simulink model "OpenFAST_ROSCO_LDP_FFP_with_FFIPC"  (R2024b)
settings: Solver=ode4  StartTime=0.0  StopTime=TMax  FixedStep=DT  RelTol=1e-3
values from neighbouring files (symbols this model uses):
  IPC = []    [HVFF_SimulinkFFIPC.m]    (also in RunExample_Simulink.m; VerticalGain_BruteForce.m)
  P = ReadWrite_FAST(fast)    [HVFF_SimulinkFFIPC.m]    (also in RunExample_Simulink.m; VerticalGain_BruteForce.m)
  verticalShear = 0.02    [HVFF_SimulinkFFIPC.m]    (also in RunExample_Simulink.m = 0.0167; VerticalGain_BruteForce.m = 0.0167)
undefined symbols (not defined in the file or in its folder): dspblkCoreblockFVToolHelper, F, gcbh, GetFASTPar, LDP, OutList, R, simu, strmatch
libraries: simulink_extras x4, simulink x3
settings Model: LastModifiedBy=demit
settings OptimizationCC: BlockReduction=off  BooleanDataType=off
settings DebuggingCC: SaveWithParameterizedLinksMsg=none  UnderspecifiedInitializationDetection=Classic  MergeDetectMultiDrivingBlocksExec=none  SignalResolutionControl=TryResolveAllWithWarning  UnconnectedInputMsg=warning  UnconnectedOutputMsg=warning  UnconnectedLineMsg=warning
settings HardwareCC: TargetUnknown=on
settings ModelReferenceCC: EnableRefExpFcnMdlSchedulingChecks=on  PropagateSignalLabelsOutOfModel=off
settings RTWCC: GPUComputeCapability=3.5  DLArmComputeVersion=19.05

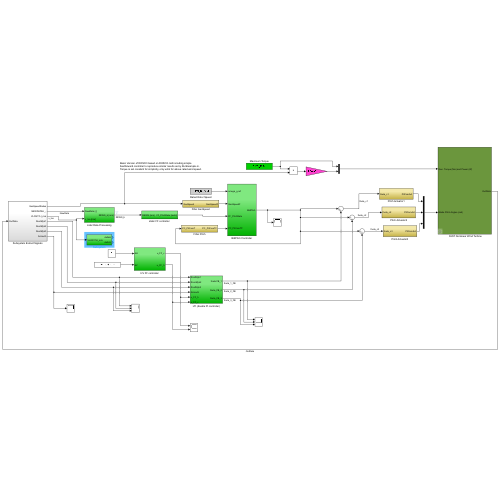
[thumbnail: Simulink's stored preview of the top-level diagram]
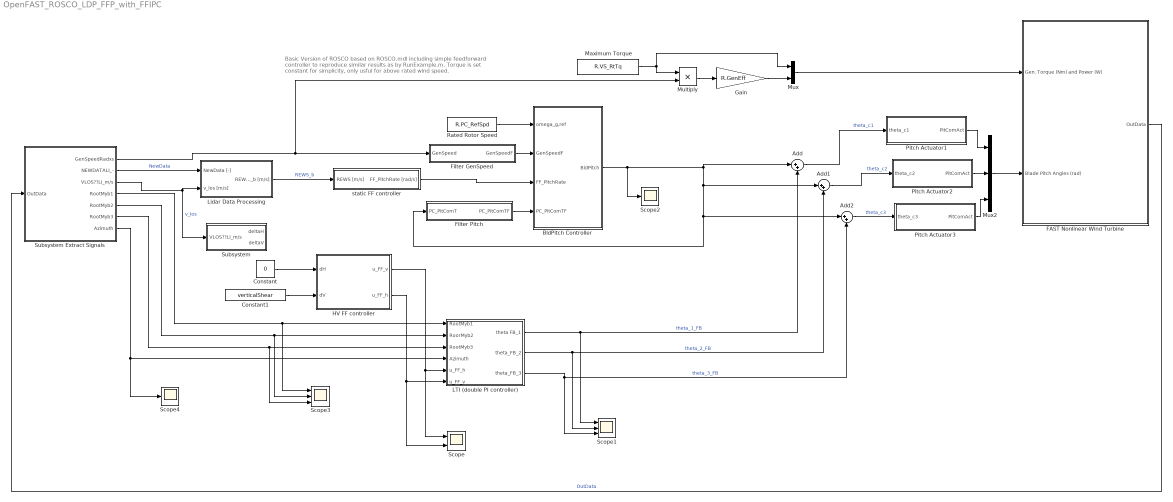
== system OpenFAST_ROSCO_LDP_FFP_with_FFIPC ==
  note: Basic Version of ROSCO based on ROSCO.mdl including simple feedforward controller to reproduce similar results as by RunExample.m.
      | Torque is set constant for simplicity, only usful for above rated wind speed.
  "  FAST Nonlinear Wind Turbine" : Subsystem  mask(FAST Nonlinear Wind Turbine){}
      mask help: This block contains the FAST S-Function.
      mask init:
      | clear FAST_SFunc
  Add : Sum  Inputs=|++
  Add1 : Sum  Inputs=|++
  Add2 : Sum  Inputs=|++
  BldPitch Controller : Subsystem
  Constant : Constant  Value=0
  Constant1 : Constant  Value=verticalShear
  Filter GenSpeed : Subsystem
  Filter Pitch : Subsystem
  Gain : Gain  Gain=R.GenEff
  HV FF controller : Subsystem
  LTI (double PI controller) : Subsystem
  Lidar Data Processing : Subsystem
  Maximum Torque : Constant  Value=R.VS_RtTq
  Multiply : Product
  Mux : Mux  Inputs=2
  Mux2 : Mux  Inputs=3
  Pitch Actuator1 : Subsystem
  Pitch Actuator2 : Subsystem
  Pitch Actuator3 : Subsystem
  Rated Rotor Speed : Constant  Value=R.PC_RefSpd
  Scope : Scope  NumInputPorts=2
  Scope1 : Scope  NumInputPorts=3
  Scope2 : Scope
  Scope3 : Scope  NumInputPorts=3
  Scope4 : Scope
  Subsystem : Subsystem
  Subsystem Extract Signals : Subsystem
  "static FF controller " : Subsystem
  wires:
  Mux2/1 -> "  FAST Nonlinear Wind Turbine"/2(Blade Pitch Angles (rad))
  BldPitch Controller/1(BldPitch) -> Scope2/1, Add/1, Add1/1, Add2/1, Filter Pitch/1(PC_PitComT)
  Rated Rotor Speed/1 -> BldPitch Controller/1(omega_g,ref)
  Subsystem Extract Signals/1(GenSpeedRadxs) -> Filter GenSpeed/1(GenSpeed), Multiply/2
  Maximum Torque/1 -> Mux/1, Multiply/1
  Filter GenSpeed/1(GenSpeedF) -> BldPitch Controller/2(GenSpeedF)
  Gain/1 -> Mux/2
  Mux/1 -> "  FAST Nonlinear Wind Turbine"/1(Gen. Torque (Nm) and Power (W))
  Multiply/1 -> Gain/1
  "  FAST Nonlinear Wind Turbine"/1(OutData) -> Subsystem Extract Signals/1(OutData)  "OutData"
  Filter Pitch/1(PC_PitComTF) -> BldPitch Controller/4(PC_PitComTF)
  Pitch Actuator1/1(PitComAct) -> Mux2/1
  "static FF controller "/1(FF_PitchRate [rad/s]) -> BldPitch Controller/3(FF_PitchRate)
  Subsystem Extract Signals/3(VLOS??LI_m/s) -> Subsystem/1(VLOS??LI_m/s), Lidar Data Processing/2(v_los [m/s])  "v_los"
  Subsystem Extract Signals/2(NEWDATALI_-) -> Lidar Data Processing/1(NewData [-])  "NewData"
  Subsystem Extract Signals/4(RootMyb1) -> Scope3/1, LTI (double PI controller)/1(RootMyb1)
  Subsystem Extract Signals/5(RootMyb2) -> Scope3/2, LTI (double PI controller)/2(RoorMyb2)
  Subsystem Extract Signals/6(RootMyb3) -> Scope3/3, LTI (double PI controller)/3(RootMyb3)
  Add/1 -> Pitch Actuator1/1(theta_c1)  "theta_c1"
  Add1/1 -> Pitch Actuator2/1(theta_c2)  "theta_c2"
  Pitch Actuator2/1(PitComAct) -> Mux2/2
  Add2/1 -> Pitch Actuator3/1(theta_c3)  "theta_c3"
  Pitch Actuator3/1(PitComAct) -> Mux2/3
  Subsystem Extract Signals/7(Azimuth) -> Scope4/1, LTI (double PI controller)/4(Azimuth)
  LTI (double PI controller)/1(theta FB_1) -> Add/2, Scope1/1  "theta_1_FB"
  LTI (double PI controller)/2(theta_FB_2) -> Add1/2, Scope1/2  "theta_2_FB"
  LTI (double PI controller)/3(theta_FB_3) -> Add2/2, Scope1/3  "theta_3_FB"
  Constant/1 -> HV FF controller/1(dH)
  Constant1/1 -> HV FF controller/2(dV)
  Lidar Data Processing/1(REWS_b [m/s]) -> "static FF controller "/1(REWS [m/s])  "REWS_b"
  HV FF controller/1(u_FF_v) -> Scope/1, LTI (double PI controller)/5(u_FF_h)
  HV FF controller/2(u_FF_h) -> Scope/2, LTI (double PI controller)/6(u_FF_v)

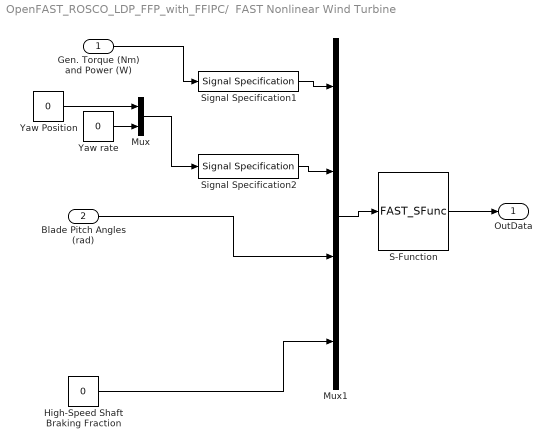
== system OpenFAST_ROSCO_LDP_FFP_with_FFIPC/  FAST Nonlinear Wind Turbine ==
  Gen. Torque (Nm) and Power (W) : Inport
  Blade Pitch Angles (rad) : Inport  Port=2
  High-Speed Shaft Braking Fraction : Constant  Value=0
  Mux : Mux  Inputs=2
  Mux1 : Mux
  S-Function : S-Function  FunctionName=FAST_SFunc  Parameters=FAST_InputFileName, TMax, 0  SFunctionDeploymentMode=off  EnableBusSupport=off
  Signal Specification1 : SignalSpecification  OutDataTypeStr=double  Dimensions=2
  Signal Specification2 : SignalSpecification  OutDataTypeStr=double  Dimensions=2
  Yaw Position : Constant  Value=0
  Yaw rate : Constant  Value=0
  OutData : Outport
  wires:
  Gen. Torque (Nm) and Power (W)/1 -> Signal Specification1/1
  S-Function/1 -> OutData/1
  Mux1/1 -> S-Function/1
  Blade Pitch Angles (rad)/1 -> Mux1/3
  Signal Specification1/1 -> Mux1/1
  Signal Specification2/1 -> Mux1/2
  High-Speed Shaft Braking Fraction/1 -> Mux1/4
  Yaw rate/1 -> Mux/2
  Mux/1 -> Signal Specification2/1
  Yaw Position/1 -> Mux/1

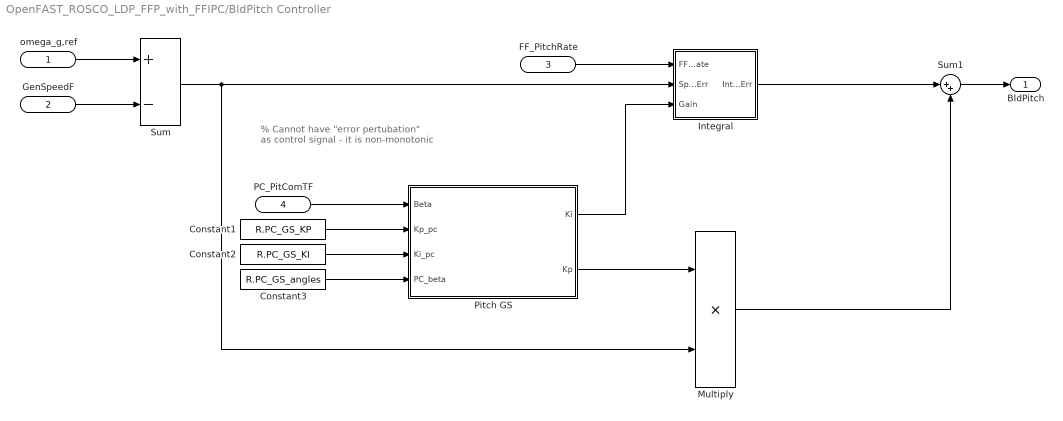
== system OpenFAST_ROSCO_LDP_FFP_with_FFIPC/BldPitch Controller ==
  note: % Cannot have "error pertubation" as control signal
      | - it is non-monotonic
  omega_g,ref : Inport
  GenSpeedF : Inport  Port=2
  FF_PitchRate : Inport  Port=3
  PC_PitComTF : Inport  Port=4
  Constant1 : Constant  Value=R.PC_GS_KP
  Constant2 : Constant  Value=R.PC_GS_KI
  Constant3 : Constant  Value=R.PC_GS_angles
  Integral : Subsystem
  Multiply : Product
  Pitch GS : MATLAB Function  TreatAsAtomicUnit=on
  Sum : Sum  Inputs=+-
  Sum1 : Sum  Inputs=|++
  BldPitch : Outport  VectorParamsAs1DForOutWhenUnconnected=off
  wires:
  Pitch GS/1(Ki) -> Integral/3(Gain)
  omega_g,ref/1 -> Sum/1
  GenSpeedF/1 -> Sum/2
  Constant1/1 -> Pitch GS/2(Kp_pc)
  Constant2/1 -> Pitch GS/3(Ki_pc)
  Constant3/1 -> Pitch GS/4(PC_beta)
  Sum/1 -> Multiply/2, Integral/2(SpeedErr)
  Multiply/1 -> Sum1/2
  Integral/1(IntSpdErr) -> Sum1/1
  Sum1/1 -> BldPitch/1
  PC_PitComTF/1 -> Pitch GS/1(Beta)
  FF_PitchRate/1 -> Integral/1(FF_PitchRate)
  Pitch GS/2(Kp) -> Multiply/1

== system OpenFAST_ROSCO_LDP_FFP_with_FFIPC/Filter GenSpeed ==
  GenSpeed : Inport
  Discrete Filter : DiscreteFilter  Numerator=F.HSS.b  Denominator=F.HSS.a  InitialStates=R.PC_RefSpd/(sum(F.HSS.a(2:end))+1)
  GenSpeedF : Outport  VectorParamsAs1DForOutWhenUnconnected=off
  wires:
  Discrete Filter/1 -> GenSpeedF/1
  GenSpeed/1 -> Discrete Filter/1

== system OpenFAST_ROSCO_LDP_FFP_with_FFIPC/Filter Pitch ==
  PC_PitComT : Inport
  Discrete Filter : DiscreteFilter  LoadFcn=dspblkCoreblockFVToolHelper(gcbh,'load');  Numerator=F.P.b  Denominator=F.P.a
      settings: CopyFcn=dspblkCoreblockFVToolHelper(gcbh,'copy');  DeleteFcn=dspblkCoreblockFVToolHelper(gcbh,'close');  ModelCloseFcn=dspblkCoreblockFVToolHelper(gcbh,'close');  PreSaveFcn=dspblkCoreblockFVToolHelper(gcbh,'presave');  PostSaveFcn=dspblkCoreblockFVToolHelper(gcbh,'postsave');  CloseFcn=dspblkCoreblockFVToolHelper(gcbh,'close');
  Unit Delay : UnitDelay  SampleTime=-1  HasFrameUpgradeWarning=on
  PC_PitComTF : Outport  VectorParamsAs1DForOutWhenUnconnected=off
  wires:
  PC_PitComT/1 -> Unit Delay/1
  Discrete Filter/1 -> PC_PitComTF/1
  Unit Delay/1 -> Discrete Filter/1

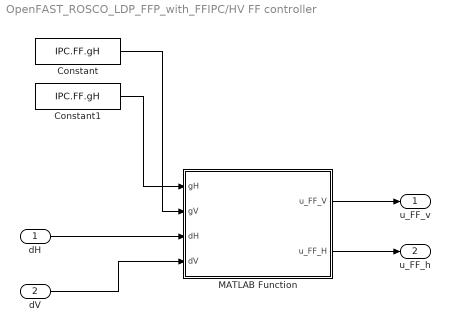
== system OpenFAST_ROSCO_LDP_FFP_with_FFIPC/HV FF controller ==
  dH : Inport
  dV : Inport  Port=2
  Constant : Constant  Value=IPC.FF.gH
  Constant1 : Constant  Value=IPC.FF.gH
  MATLAB Function : MATLAB Function  TreatAsAtomicUnit=on
  u_FF_v : Outport
  u_FF_h : Outport  Port=2
  wires:
  dH/1 -> MATLAB Function/3(dH)
  dV/1 -> MATLAB Function/4(dV)
  Constant1/1 -> MATLAB Function/1(gH)
  Constant/1 -> MATLAB Function/2(gV)
  MATLAB Function/2(u_FF_H) -> u_FF_h/1
  MATLAB Function/1(u_FF_V) -> u_FF_v/1

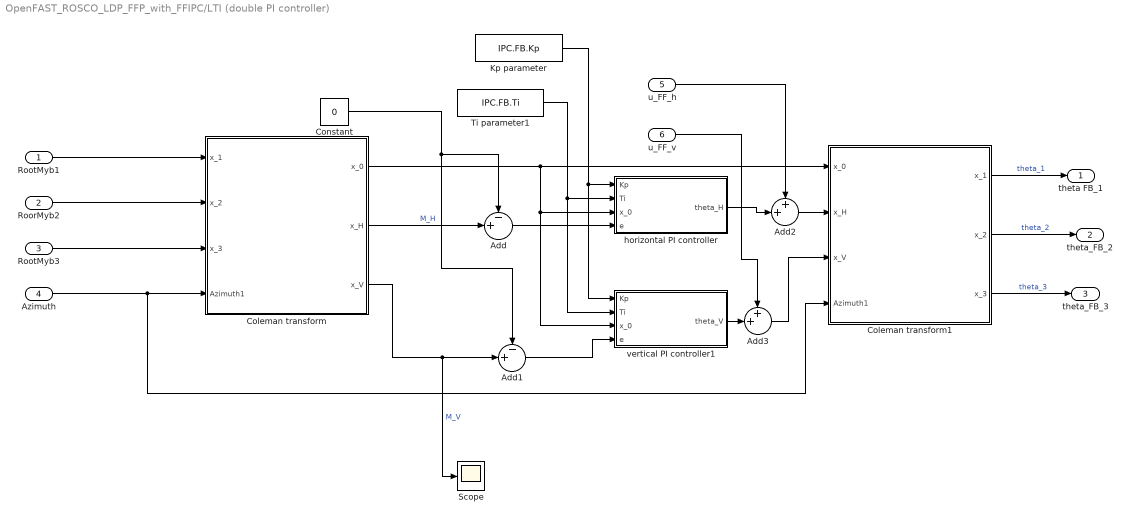
== system OpenFAST_ROSCO_LDP_FFP_with_FFIPC/LTI (double PI controller) ==
  RootMyb1 : Inport
  RoorMyb2 : Inport  Port=2
  RootMyb3 : Inport  Port=3
  Azimuth : Inport  Port=4
  u_FF_h : Inport  Port=5
  u_FF_v : Inport  Port=6
  Add : Sum  Inputs=-+|
  Add1 : Sum  Inputs=-+|
  Add2 : Sum  Inputs=++|
  Add3 : Sum  Inputs=++|
  Coleman transform : MATLAB Function  TreatAsAtomicUnit=on
  Coleman transform1 : MATLAB Function  TreatAsAtomicUnit=on
  Constant : Constant  Value=0
  Kp parameter : Constant  Value=IPC.FB.Kp
  Scope : Scope
  Ti parameter1 : Constant  Value=IPC.FB.Ti
  horizontal PI controller : Subsystem
  vertical PI controller1 : Subsystem
  theta FB_1 : Outport
  theta_FB_2 : Outport  Port=2
  theta_FB_3 : Outport  Port=3
  wires:
  RootMyb1/1 -> Coleman transform/1(x_1)
  RootMyb3/1 -> Coleman transform/3(x_3)
  Azimuth/1 -> Coleman transform1/4(Azimuth1), Coleman transform/4(Azimuth1)
  Coleman transform/1(x_0) -> vertical PI controller1/3(x_0), horizontal PI controller/3(x_0), Coleman transform1/1(x_0)
  Coleman transform/2(x_H) -> Add/2  "M_H"
  Constant/1 -> Add/1, Add1/1
  Add/1 -> horizontal PI controller/4(e)
  Coleman transform/3(x_V) -> Scope/1, Add1/2  "M_V"
  Add1/1 -> vertical PI controller1/4(e)
  Ti parameter1/1 -> vertical PI controller1/2(Ti), horizontal PI controller/2(Ti)
  Kp parameter/1 -> vertical PI controller1/1(Kp), horizontal PI controller/1(Kp)
  RoorMyb2/1 -> Coleman transform/2(x_2)
  Coleman transform1/3(x_3) -> theta_FB_3/1  "theta_3"
  Coleman transform1/2(x_2) -> theta_FB_2/1  "theta_2"
  Coleman transform1/1(x_1) -> theta FB_1/1  "theta_1"
  u_FF_v/1 -> Add3/1
  vertical PI controller1/1(theta_V) -> Add3/2
  Add3/1 -> Coleman transform1/3(x_V)
  horizontal PI controller/1(theta_H) -> Add2/2
  Add2/1 -> Coleman transform1/2(x_H)
  u_FF_h/1 -> Add2/1

== system OpenFAST_ROSCO_LDP_FFP_with_FFIPC/Lidar Data Processing ==
  NewData [-] : Inport
  v_los [m/s] : Inport  Port=2
  Buffer : Subsystem
  LPFilter : Subsystem
  WindFieldReconstruction : Subsystem
  REWS_b [m/s] : Outport  VectorParamsAs1DForOutWhenUnconnected=off
  wires:
  v_los [m/s]/1 -> WindFieldReconstruction/1(v_los [m/s])  "v_los"
  NewData [-]/1 -> WindFieldReconstruction/Enable
  Buffer/1(REWS_b [m/s]) -> REWS_b [m/s]/1  "REWS_b"
  WindFieldReconstruction/1(REWS [m/s]) -> LPFilter/1(REWS [m/s])  "REWS"
  LPFilter/1(REWS_f [m/s]) -> Buffer/1(REWS_f [m/s])  "REWS_f"

== system OpenFAST_ROSCO_LDP_FFP_with_FFIPC/Pitch Actuator1 ==
  theta_c1 : Inport
  Discrete Filter : DiscreteFilter  LoadFcn=dspblkCoreblockFVToolHelper(gcbh,'load');  Numerator=F.F_PitchAct.b  Denominator=F.F_PitchAct.a  InitialStates=GetFASTPar(P.EDP,'BlPitch(1)')/180*pi/(sum(F.F_PitchAct.a(2:end))+1)
      settings: CopyFcn=dspblkCoreblockFVToolHelper(gcbh,'copy');  DeleteFcn=dspblkCoreblockFVToolHelper(gcbh,'close');  ModelCloseFcn=dspblkCoreblockFVToolHelper(gcbh,'close');  PreSaveFcn=dspblkCoreblockFVToolHelper(gcbh,'presave');  PostSaveFcn=dspblkCoreblockFVToolHelper(gcbh,'postsave');  CloseFcn=dspblkCoreblockFVToolHelper(gcbh,'close');
  PitComAct : Outport  VectorParamsAs1DForOutWhenUnconnected=off
  wires:
  theta_c1/1 -> Discrete Filter/1
  Discrete Filter/1 -> PitComAct/1

== system OpenFAST_ROSCO_LDP_FFP_with_FFIPC/Pitch Actuator2 ==
  theta_c2 : Inport
  Discrete Filter : DiscreteFilter  LoadFcn=dspblkCoreblockFVToolHelper(gcbh,'load');  Numerator=F.F_PitchAct.b  Denominator=F.F_PitchAct.a  InitialStates=GetFASTPar(P.EDP,'BlPitch(1)')/180*pi/(sum(F.F_PitchAct.a(2:end))+1)
      settings: CopyFcn=dspblkCoreblockFVToolHelper(gcbh,'copy');  DeleteFcn=dspblkCoreblockFVToolHelper(gcbh,'close');  ModelCloseFcn=dspblkCoreblockFVToolHelper(gcbh,'close');  PreSaveFcn=dspblkCoreblockFVToolHelper(gcbh,'presave');  PostSaveFcn=dspblkCoreblockFVToolHelper(gcbh,'postsave');  CloseFcn=dspblkCoreblockFVToolHelper(gcbh,'close');
  PitComAct : Outport  VectorParamsAs1DForOutWhenUnconnected=off
  wires:
  theta_c2/1 -> Discrete Filter/1
  Discrete Filter/1 -> PitComAct/1

== system OpenFAST_ROSCO_LDP_FFP_with_FFIPC/Pitch Actuator3 ==
  theta_c3 : Inport
  Discrete Filter : DiscreteFilter  LoadFcn=dspblkCoreblockFVToolHelper(gcbh,'load');  Numerator=F.F_PitchAct.b  Denominator=F.F_PitchAct.a  InitialStates=GetFASTPar(P.EDP,'BlPitch(1)')/180*pi/(sum(F.F_PitchAct.a(2:end))+1)
      settings: CopyFcn=dspblkCoreblockFVToolHelper(gcbh,'copy');  DeleteFcn=dspblkCoreblockFVToolHelper(gcbh,'close');  ModelCloseFcn=dspblkCoreblockFVToolHelper(gcbh,'close');  PreSaveFcn=dspblkCoreblockFVToolHelper(gcbh,'presave');  PostSaveFcn=dspblkCoreblockFVToolHelper(gcbh,'postsave');  CloseFcn=dspblkCoreblockFVToolHelper(gcbh,'close');
  PitComAct : Outport  VectorParamsAs1DForOutWhenUnconnected=off
  wires:
  theta_c3/1 -> Discrete Filter/1
  Discrete Filter/1 -> PitComAct/1

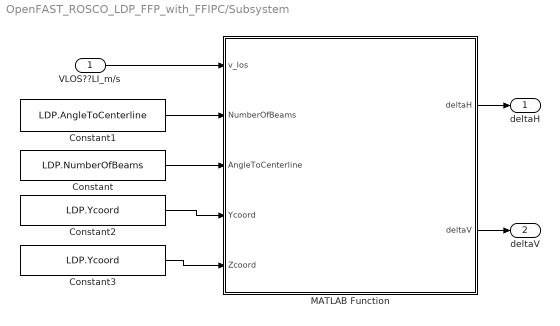
== system OpenFAST_ROSCO_LDP_FFP_with_FFIPC/Subsystem ==
  VLOS??LI_m/s : Inport
  Constant : Constant  Value=LDP.NumberOfBeams
  Constant1 : Constant  Value=LDP.AngleToCenterline
  Constant2 : Constant  Value=LDP.Ycoord
  Constant3 : Constant  Value=LDP.Ycoord
  MATLAB Function : MATLAB Function  TreatAsAtomicUnit=on
  deltaH : Outport
  deltaV : Outport  Port=2
  wires:
  VLOS??LI_m/s/1 -> MATLAB Function/1(v_los)
  MATLAB Function/1(deltaH) -> deltaH/1
  Constant/1 -> MATLAB Function/3(AngleToCenterline)
  Constant1/1 -> MATLAB Function/2(NumberOfBeams)
  MATLAB Function/2(deltaV) -> deltaV/1
  Constant2/1 -> MATLAB Function/4(Ycoord)
  Constant3/1 -> MATLAB Function/5(Zcoord)

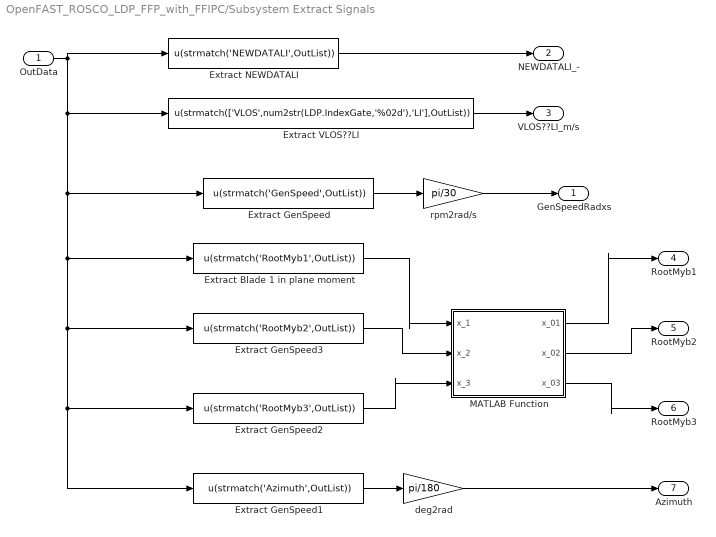
== system OpenFAST_ROSCO_LDP_FFP_with_FFIPC/Subsystem Extract Signals ==
  OutData : Inport
  Extract Blade 1 in plane moment : Fcn  Expr=u(strmatch('RootMyb1',OutList))
  Extract GenSpeed : Fcn  Expr=u(strmatch('GenSpeed',OutList))
  Extract GenSpeed1 : Fcn  Expr=u(strmatch('Azimuth',OutList))
  Extract GenSpeed2 : Fcn  Expr=u(strmatch('RootMyb3',OutList))
  Extract GenSpeed3 : Fcn  Expr=u(strmatch('RootMyb2',OutList))
  Extract NEWDATALI : Fcn  Expr=u(strmatch('NEWDATALI',OutList))
  Extract VLOS??LI : Fcn  Expr=u(strmatch(['VLOS',num2str(LDP.IndexGate,'%02d'),'LI'],OutList))
  MATLAB Function : MATLAB Function  TreatAsAtomicUnit=on
  deg2rad : Gain  Gain=pi/180
  rpm2rad/s : Gain  Gain=pi/30
  GenSpeedRadxs : Outport
  NEWDATALI_- : Outport  Port=2  VectorParamsAs1DForOutWhenUnconnected=off
  VLOS??LI_m/s : Outport  Port=3  VectorParamsAs1DForOutWhenUnconnected=off
  RootMyb1 : Outport  Port=4
  RootMyb2 : Outport  Port=5
  RootMyb3 : Outport  Port=6
  Azimuth : Outport  Port=7
  wires:
  Extract GenSpeed/1 -> rpm2rad/s/1
  Extract VLOS??LI/1 -> VLOS??LI_m/s/1
  Extract NEWDATALI/1 -> NEWDATALI_-/1
  OutData/1 -> Extract GenSpeed1/1, Extract GenSpeed2/1, Extract GenSpeed3/1, Extract Blade 1 in plane moment/1, Extract GenSpeed/1, Extract VLOS??LI/1, Extract NEWDATALI/1
  Extract Blade 1 in plane moment/1 -> MATLAB Function/1(x_1)
  Extract GenSpeed3/1 -> MATLAB Function/2(x_2)
  Extract GenSpeed2/1 -> MATLAB Function/3(x_3)
  MATLAB Function/1(x_01) -> RootMyb1/1
  MATLAB Function/2(x_02) -> RootMyb2/1
  MATLAB Function/3(x_03) -> RootMyb3/1
  rpm2rad/s/1 -> GenSpeedRadxs/1
  Extract GenSpeed1/1 -> deg2rad/1
  deg2rad/1 -> Azimuth/1

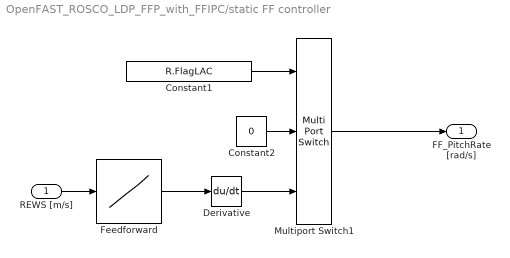
== system OpenFAST_ROSCO_LDP_FFP_with_FFIPC/static FF controller  ==
  REWS [m/s] : Inport
  Constant1 : Constant  Value=R.FlagLAC
  Constant2 : Constant  Value=0
  Derivative : Derivative
  Feedforward : Lookup_n-D  NumberOfTableDimensions=1  BreakpointsForDimension1=R.StaticWind  Table=R.StaticPitch  InternalRulePriority=Speed  RndMeth=Simplest
  Multiport Switch1 : MultiPortSwitch  DataPortOrder=Specify indices  Inputs=2  DataPortIndices={0,1}  SaturateOnIntegerOverflow=off  InputSameDT=off
  FF_PitchRate [rad/s] : Outport  VectorParamsAs1DForOutWhenUnconnected=off
  wires:
  Multiport Switch1/1 -> FF_PitchRate [rad/s]/1
  Feedforward/1 -> Derivative/1
  Constant1/1 -> Multiport Switch1/1
  Constant2/1 -> Multiport Switch1/2
  REWS [m/s]/1 -> Feedforward/1
  Derivative/1 -> Multiport Switch1/3

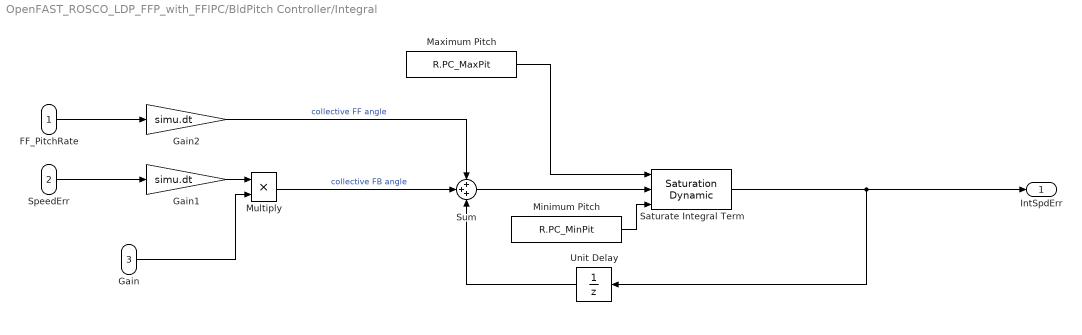
== system OpenFAST_ROSCO_LDP_FFP_with_FFIPC/BldPitch Controller/Integral ==
  FF_PitchRate : Inport
  SpeedErr : Inport  Port=2
  Gain : Inport  Port=3
  Gain1 : Gain  Gain=simu.dt
  Gain2 : Gain  Gain=simu.dt
  Maximum Pitch : Constant  Value=R.PC_MaxPit
  Minimum Pitch : Constant  Value=R.PC_MinPit
  Multiply : Product
  Saturate Integral Term : simulink/Discontinuities/Saturation Dynamic  OutMin=[]  OutMax=[]  OutDataTypeStr=Inherit: Same as second input  OutDataType=fixdt(1, 16)  OutScaling=2^-10  RndMeth=Nearest  DoSatur=off
  Sum : Sum  Inputs=+++
  Unit Delay : UnitDelay  InitialCondition=GetFASTPar(P.EDP,'BlPitch(1)')/180*pi  SampleTime=-1  HasFrameUpgradeWarning=on
  IntSpdErr : Outport  VectorParamsAs1DForOutWhenUnconnected=off
  wires:
  Maximum Pitch/1 -> Saturate Integral Term/1
  Sum/1 -> Saturate Integral Term/2
  SpeedErr/1 -> Gain1/1
  Gain/1 -> Multiply/2
  Saturate Integral Term/1 -> IntSpdErr/1, Unit Delay/1
  Gain1/1 -> Multiply/1
  Minimum Pitch/1 -> Saturate Integral Term/3
  Unit Delay/1 -> Sum/3
  Multiply/1 -> Sum/2  "collective FB angle"
  Gain2/1 -> Sum/1  "collective FF angle"
  FF_PitchRate/1 -> Gain2/1

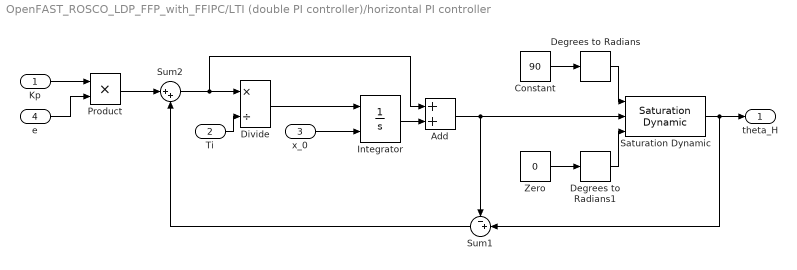
== system OpenFAST_ROSCO_LDP_FFP_with_FFIPC/LTI (double PI controller)/horizontal PI controller ==
  Kp : Inport
  Ti : Inport  Port=2
  x_0 : Inport  Port=3
  e : Inport  Port=4
  Add : Sum
  Constant : Constant  Value=90
  Degrees to Radians : simulink_extras/Transformations/Degrees to Radians
  Degrees to Radians1 : simulink_extras/Transformations/Degrees to Radians
  Divide : Product  Inputs=*/
  Integrator : Integrator  InitialConditionSource=external
  Product : Product
  Saturation Dynamic : simulink/Discontinuities/Saturation Dynamic  OutMin=[]  OutMax=[]  OutDataTypeStr=Inherit: Same as second input  OutDataType=fixdt(1, 16)  OutScaling=2^-10  DoSatur=off
  Sum1 : Sum  Inputs=-+|
  Sum2 : Sum  Inputs=|++
  Zero : Constant  Value=0  OutDataTypeStr=Inherit: Inherit via back propagation
  theta_H : Outport
  wires:
  Kp/1 -> Product/1
  e/1 -> Product/2
  Product/1 -> Sum2/1
  Ti/1 -> Divide/2
  x_0/1 -> Integrator/2
  Divide/1 -> Integrator/1
  Integrator/1 -> Add/2
  Add/1 -> Sum1/1, Saturation Dynamic/2
  Saturation Dynamic/1 -> Sum1/2, theta_H/1
  Degrees to Radians1/1 -> Saturation Dynamic/3
  Zero/1 -> Degrees to Radians1/1
  Degrees to Radians/1 -> Saturation Dynamic/1
  Constant/1 -> Degrees to Radians/1
  Sum1/1 -> Sum2/2
  Sum2/1 -> Add/1, Divide/1

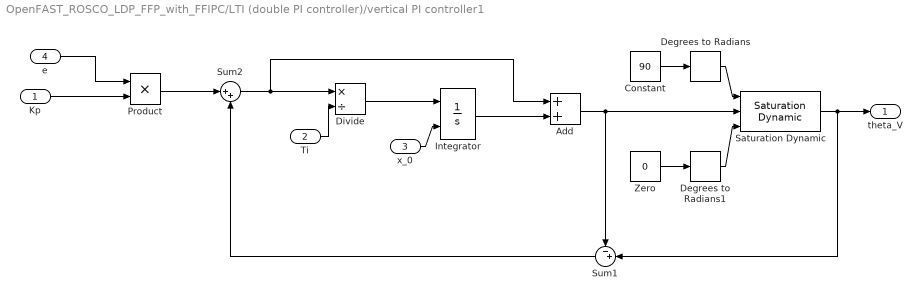
== system OpenFAST_ROSCO_LDP_FFP_with_FFIPC/LTI (double PI controller)/vertical PI controller1 ==
  Kp : Inport
  Ti : Inport  Port=2
  x_0 : Inport  Port=3
  e : Inport  Port=4
  Add : Sum
  Constant : Constant  Value=90
  Degrees to Radians : simulink_extras/Transformations/Degrees to Radians
  Degrees to Radians1 : simulink_extras/Transformations/Degrees to Radians
  Divide : Product  Inputs=*/
  Integrator : Integrator  InitialConditionSource=external
  Product : Product
  Saturation Dynamic : simulink/Discontinuities/Saturation Dynamic  OutMin=[]  OutMax=[]  OutDataTypeStr=Inherit: Same as second input  OutDataType=fixdt(1, 16)  OutScaling=2^-10  DoSatur=off
  Sum1 : Sum  Inputs=-+|
  Sum2 : Sum  Inputs=|++
  Zero : Constant  Value=0  OutDataTypeStr=Inherit: Inherit via back propagation
  theta_V : Outport
  wires:
  e/1 -> Product/1
  Kp/1 -> Product/2
  x_0/1 -> Integrator/2
  Ti/1 -> Divide/2
  Divide/1 -> Integrator/1
  Integrator/1 -> Add/2
  Zero/1 -> Degrees to Radians1/1
  Constant/1 -> Degrees to Radians/1
  Degrees to Radians1/1 -> Saturation Dynamic/3
  Degrees to Radians/1 -> Saturation Dynamic/1
  Add/1 -> Sum1/1, Saturation Dynamic/2
  Saturation Dynamic/1 -> Sum1/2, theta_V/1
  Sum1/1 -> Sum2/2
  Product/1 -> Sum2/1
  Sum2/1 -> Add/1, Divide/1

== system OpenFAST_ROSCO_LDP_FFP_with_FFIPC/Lidar Data Processing/Buffer ==
  REWS_f [m/s] : Inport
  Constant1 : Constant  Value=LDP.T_buffer
  Constant2 : Constant  Value=simu.dt
  MATLAB Function : MATLAB Function  TreatAsAtomicUnit=on
  REWS_b [m/s] : Outport  VectorParamsAs1DForOutWhenUnconnected=off
  wires:
  Constant1/1 -> MATLAB Function/3(T_buffer)
  Constant2/1 -> MATLAB Function/2(DT)
  REWS_f [m/s]/1 -> MATLAB Function/1(REWS)
  MATLAB Function/1(REWS_b) -> REWS_b [m/s]/1

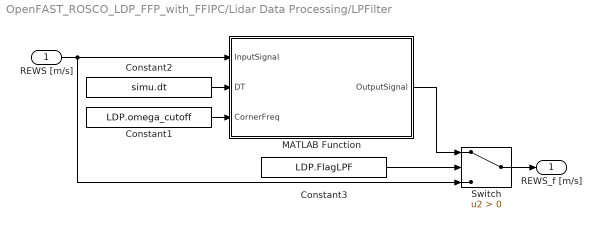
== system OpenFAST_ROSCO_LDP_FFP_with_FFIPC/Lidar Data Processing/LPFilter ==
  REWS [m/s] : Inport
  Constant1 : Constant  Value=LDP.omega_cutoff
  Constant2 : Constant  Value=simu.dt
  Constant3 : Constant  Value=LDP.FlagLPF
  MATLAB Function : MATLAB Function  TreatAsAtomicUnit=on
  Switch : Switch  Criteria=u2 > Threshold  SaturateOnIntegerOverflow=off  InputSameDT=off
  REWS_f [m/s] : Outport  VectorParamsAs1DForOutWhenUnconnected=off
  wires:
  REWS [m/s]/1 -> MATLAB Function/1(InputSignal), Switch/3
  Constant2/1 -> MATLAB Function/2(DT)
  Constant1/1 -> MATLAB Function/3(CornerFreq)
  Switch/1 -> REWS_f [m/s]/1
  Constant3/1 -> Switch/2
  MATLAB Function/1(OutputSignal) -> Switch/1

== system OpenFAST_ROSCO_LDP_FFP_with_FFIPC/Lidar Data Processing/WindFieldReconstruction ==
  v_los [m/s] : Inport
  Enable : EnablePort
  Constant1 : Constant  Value=LDP.AngleToCenterline
  Constant2 : Constant  Value=LDP.NumberOfBeams
  MATLAB Function : MATLAB Function  TreatAsAtomicUnit=on
  REWS [m/s] : Outport  VectorParamsAs1DForOutWhenUnconnected=off
  wires:
  MATLAB Function/1(REWS) -> REWS [m/s]/1
  v_los [m/s]/1 -> MATLAB Function/1(v_los)
  Constant2/1 -> MATLAB Function/2(NumberOfBeams)
  Constant1/1 -> MATLAB Function/3(AngleToCenterline)

== matlab function OpenFAST_ROSCO_LDP_FFP_with_FFIPC/HV FF controller/MATLAB Function ==
  data: gH input; gV input; dH input; u_FF_V output; dV input; u_FF_H output
function [u_FF_V,u_FF_H] = asynchronous_ctrl(gH, gV, dH, dV)

d_ss_HV = [dH dV]';

u_ss_HV = [gH 0; 0 gV] * d_ss_HV;

u_FF_H = u_ss_HV(1);
u_FF_V = u_ss_HV(2);

end

== matlab function OpenFAST_ROSCO_LDP_FFP_with_FFIPC/Subsystem/MATLAB Function ==
  data: v_los input; deltaH output; deltaV output; NumberOfBeams input; AngleToCenterline input; Ycoord input; Zcoord input
function [deltaH,deltaV] = CalculateShears(v_los,NumberOfBeams,AngleToCenterline, Ycoord, Zcoord)

u_est = v_los/AngleToCenterline;

n = 1:NumberOfBeams/2;
deltaH_vec = zeros(n,1);
deltaV_vec = zeros(n,1);

% horizontal shear
for i = 1:n
    u_east      = u_est(i);
    u_west      = u_est(NumberOfBeams+1-i);
    y_east      = Ycoord(i);
    y_west      = Zcoord(NumberOfBeams+1-i);

    delta_u     = abs(u_west-u_east);
    deltay      = y_east-y_west;
    deltaH_vec(i) = delta_u/deltay;
    
end

% vertical shear
for i = 1:n
    u_east      = u_est(i);
    u_west      = u_est(NumberOfBeams+1-i);
    y_east      = Ycoord(i);
    y_west      = Zcoord(NumberOfBeams+1-i);

    delta_u     = abs(u_west-u_east);
    deltay      = y_east-y_west;
    deltaH_vec(i) = delta_u/deltay;
    
end


end

== matlab function OpenFAST_ROSCO_LDP_FFP_with_FFIPC/Lidar Data Processing/Buffer/MATLAB Function ==
  data: REWS input; REWS_b output; DT input; T_buffer input
function REWS_b = Buffer(REWS,DT,T_buffer)

% init REWS_f_Buffer
nBuffer = 2000; % Size of REWS_f_buffer, 25 seconds at 80 Hz  [-] 
persistent REWS_f_Buffer;
if isempty(REWS_f_Buffer)      
    REWS_f_Buffer = ones(nBuffer,1)*REWS;   
end 

% Update Buffer for estimated u component
REWS_f_Buffer    = [REWS;REWS_f_Buffer(1:nBuffer-1)];

% Index for entry at T_buffer, minimum 1, maximum nBuffer
Idx     = min( max(floor(T_buffer/DT),1) , nBuffer);
		
% Get buffered and filtered REWS from buffer
REWS_b  = REWS_f_Buffer(Idx);

end

== matlab function OpenFAST_ROSCO_LDP_FFP_with_FFIPC/Lidar Data Processing/WindFieldReconstruction/MATLAB Function ==
  data: v_los input; REWS output; NumberOfBeams input; AngleToCenterline input
function REWS = WindFieldReconstruction(v_los,NumberOfBeams,AngleToCenterline)
% matlab version of the subroutine WindFieldReconstruction in LDP_v1_Subs.f90

% init u_est_Buffer
persistent u_est_Buffer;
if isempty(u_est_Buffer)      
    u_est_Buffer = NaN(NumberOfBeams,1);   
end 

% Estimate u component assuming perfect alignment
u_est 		    = v_los/cosd(AngleToCenterline);

% Update Buffer for estimated u component
u_est_Buffer    = [u_est;u_est_Buffer(1:NumberOfBeams-1)];

% Calculate REWS from mean over all estimated u components
REWS  	        = mean(u_est_Buffer,'omitnan');

end

== matlab function OpenFAST_ROSCO_LDP_FFP_with_FFIPC/Lidar Data Processing/LPFilter/MATLAB Function ==
  data: InputSignal input; OutputSignal output; DT input; CornerFreq input
function OutputSignal = LPFilter(InputSignal,DT,CornerFreq)
% matlab version of the function LPFilter in FFP_v1_Subs.f90

% Initialization
persistent OutputSignalLast InputSignalLast;
if isempty(OutputSignalLast)      
    OutputSignalLast    = InputSignal;  
    InputSignalLast     = InputSignal;
end 

% Define coefficients 
a1          = 2 + CornerFreq*DT;
a0          = CornerFreq*DT - 2;
b1          = CornerFreq*DT;
b0          = CornerFreq*DT;

% Filter
OutputSignal = 1.0/a1 * (-a0*OutputSignalLast + b1*InputSignal + b0*InputSignalLast);

% Save signals for next time step
InputSignalLast     = InputSignal;
OutputSignalLast    = OutputSignal;
end

== matlab function OpenFAST_ROSCO_LDP_FFP_with_FFIPC/LTI (double PI controller)/Coleman transform ==
  data: x_0 output; x_1 input; x_2 input; x_3 input; x_H output; Azimuth1 input; x_V output
function [x_0,x_H,x_V] = Coleman_TR(x_1, x_2, x_3, Azimuth1)

Azimuth2 = Azimuth1+2/3*pi;
Azimuth3 = Azimuth2+2/3*pi;

% Coleman transformation

x_0 = 0;
x_H = x_0 + 2/3*(cos(Azimuth1)*x_1+cos(Azimuth2)*x_2+cos(Azimuth3)*x_3);
x_V = x_0 + 2/3*(sin(Azimuth1)*x_1+sin(Azimuth2)*x_2+sin(Azimuth3)*x_3);
end

== matlab function OpenFAST_ROSCO_LDP_FFP_with_FFIPC/Subsystem Extract Signals/MATLAB Function ==
  data: x_1 input; x_01 output; x_2 input; x_3 input; x_02 output; x_03 output
function [x_01,x_02,x_03] = detrending(x_1, x_2, x_3)

% removing the average
x_m = (x_1+x_2+x_3)/3;

x_01 = x_1-x_m;
x_02 = x_2-x_m;
x_03 = x_3-x_m;

end

== matlab function OpenFAST_ROSCO_LDP_FFP_with_FFIPC/BldPitch Controller/Pitch GS ==
  data: Ki output size=1; Beta input; Kp_pc input; Kp output size=1; Ki_pc input; PC_beta input
 function [Ki, Kp] = GainSchedule(Beta, Kp_pc, Ki_pc,  PC_beta)

% This function calculates the current gains for a Collective Blade Pitch 
% controller
%
% Inputs: v - Current wind speed estimate, m/s.
%         ContParam - Structure of control parameters, output from
%                     ControlParameters.m
%
% Outputs: Kp - Proportional Gain
%          Ki - Integral Gain
%
% Nikhar Abbas - May 2019


%% Linear Gain Schedule
% pKp_pc = ContParam.GS.pKp_pc;
% pKi_pc = ContParam.GS.pKi_pc;
% 
% %%
% Kp = pKp_pc(1)*Beta + pKp_pc(2);
% Ki = pKi_pc(1)*Beta + pKi_pc(2);
% % Kp = pKp_pc(1)*v + pKp_pc(2)
% % Ki = pKi_pc(1)*v + pKi_pc(2);
% 
% Kpmax = pKp_pc(1)*15*pi/180 + pKp_pc(2);
% Kimax = pKi_pc(1)*15*pi/180 + pKi_pc(2);
% 
% Kp = min(Kp, Kpmax);
% Ki = min(Ki,Kimax);

%% nonlinear Gain Schedule
% Kp_pc   = R.PC_GS_KP;
% Ki_pc   = R.PC_GS_KI;
% PC_beta = R.PC_GS_angles;

beta    = max(min(Beta,PC_beta(end)), PC_beta(1));

% gains
Kp      = interp1(PC_beta,Kp_pc, beta);
Ki      = interp1(PC_beta,Ki_pc, beta);



end

== matlab function OpenFAST_ROSCO_LDP_FFP_with_FFIPC/LTI (double PI controller)/Coleman transform1 ==
  data: x_1 output; x_0 input; x_H input; x_V input; x_2 output; Azimuth1 input; x_3 output
function [x_1,x_2,x_3] = Coleman_TR(x_0, x_H, x_V, Azimuth1)

Azimuth2 = Azimuth1+2/3*pi;
Azimuth3 = Azimuth2+2/3*pi;

% Coleman transformation

x_1 = x_0 + (x_V*cos(Azimuth1)+x_H*sin(Azimuth1)); % Dummy
x_2 = x_0 + (x_V*cos(Azimuth2)+x_H*sin(Azimuth2)); % Dummy
x_3 = x_0 + (x_V*cos(Azimuth3)+x_H*sin(Azimuth3)); % Dummy   

end
